simulink model "IEEE14_case"  (R2024b)
settings: Solver=FixedStepAuto  StartTime=0  StopTime=2  FixedStep=1e-7  RelTol=1e-3
values from neighbouring files (symbols this model uses):
  GFL_15_Bva = 0.009    [IEEE14_parameters.m]
  GFL_15_C_bus_pu = 7.179419    [IEEE14_parameters.m]
  GFL_15_f0 = 60    [IEEE14_parameters.m]
  GFL_15_I_id = 691.26967    [IEEE14_parameters.m]
  GFL_15_I_iq = 691.26967    [IEEE14_parameters.m]
  GFL_15_I_od = 45.2207    [IEEE14_parameters.m]
  GFL_15_I_oq = 45.2207    [IEEE14_parameters.m]
  GFL_15_I_pll = 0.78    [IEEE14_parameters.m]
  GFL_15_Kdi = 0.09    [IEEE14_parameters.m]
  GFL_15_Kdo = 0.9    [IEEE14_parameters.m]
  GFL_15_Kqi = 0.09    [IEEE14_parameters.m]
  GFL_15_Kqo = 0.9    [IEEE14_parameters.m]
  GFL_15_Lg_pu = 0.631447    [IEEE14_parameters.m]
  GFL_15_mode = 1    [IEEE14_parameters.m]
  GFL_15_P_id = 3.7166    [IEEE14_parameters.m]
  GFL_15_P_iq = 3.7166    [IEEE14_parameters.m]
  GFL_15_P_od = 0.4798    [IEEE14_parameters.m]
  GFL_15_P_oq = 0.4798    [IEEE14_parameters.m]
  GFL_15_P_pll = 290.42    [IEEE14_parameters.m]
  GFL_15_Qe_ref = 0.2    [IEEE14_parameters.m]
  GFL_15_Rg_pu = 0.024016    [IEEE14_parameters.m]
  GFL_15_Sbase = 1.000000e+4    (= 10000)    [IEEE14_parameters.m]
  GFL_15_Tdi = 0.01    [IEEE14_parameters.m]
  GFL_15_Tdo = 0.2    [IEEE14_parameters.m]
  GFL_15_Tqi = 0.01    [IEEE14_parameters.m]
  GFL_15_Tqo = 0.2    [IEEE14_parameters.m]
  GFL_15_Vbase = 380    [IEEE14_parameters.m]
  GFL_15_Vdc_ref = 1.011475    [IEEE14_parameters.m]
  GFL_15_Vdcbase = 700    [IEEE14_parameters.m]
  GFL_15_vq_ref = 0    [IEEE14_parameters.m]
  GFL_16_Bva = 0.002    [IEEE14_parameters.m]
  GFL_16_C_bus_pu = 7.179419    [IEEE14_parameters.m]
  GFL_16_f0 = 60    [IEEE14_parameters.m]
  GFL_16_I_id = 691.26967    [IEEE14_parameters.m]
  GFL_16_I_iq = 691.26967    [IEEE14_parameters.m]
  GFL_16_I_od = 45.2207    [IEEE14_parameters.m]
  GFL_16_I_oq = 45.2207    [IEEE14_parameters.m]
  GFL_16_I_pll = 0.78    [IEEE14_parameters.m]
  GFL_16_Kdi = 0.05    [IEEE14_parameters.m]
  GFL_16_Kdo = 0.5    [IEEE14_parameters.m]
  GFL_16_Kqi = 0.05    [IEEE14_parameters.m]
  GFL_16_Kqo = 0.5    [IEEE14_parameters.m]
  GFL_16_Lg_pu = 0.631447    [IEEE14_parameters.m]
  GFL_16_mode = 1    [IEEE14_parameters.m]
  GFL_16_P_id = 3.7166    [IEEE14_parameters.m]
  GFL_16_P_iq = 3.7166    [IEEE14_parameters.m]
  GFL_16_P_od = 0.4798    [IEEE14_parameters.m]
  GFL_16_P_oq = 0.4798    [IEEE14_parameters.m]
  GFL_16_P_pll = 290.42    [IEEE14_parameters.m]
  GFL_16_Qe_ref = 0.2    [IEEE14_parameters.m]
  GFL_16_Rg_pu = 0.024016    [IEEE14_parameters.m]
  GFL_16_Sbase = 1.000000e+4    (= 10000)    [IEEE14_parameters.m]
  GFL_16_Tdi = 0.01    [IEEE14_parameters.m]
  GFL_16_Tdo = 0.2    [IEEE14_parameters.m]
  GFL_16_Tqi = 0.01    [IEEE14_parameters.m]
  GFL_16_Tqo = 0.2    [IEEE14_parameters.m]
  GFL_16_Vbase = 380    [IEEE14_parameters.m]
  GFL_16_Vdc_ref = 1.01144    [IEEE14_parameters.m]
  GFL_16_Vdcbase = 700    [IEEE14_parameters.m]
  GFL_16_vq_ref = 0    [IEEE14_parameters.m]
  GFL_17_Bva = 0.002    [IEEE14_parameters.m]
  GFL_17_C_bus_pu = 7.179419    [IEEE14_parameters.m]
  GFL_17_f0 = 60    [IEEE14_parameters.m]
  GFL_17_I_id = 691.26967    [IEEE14_parameters.m]
  GFL_17_I_iq = 691.26967    [IEEE14_parameters.m]
  GFL_17_I_od = 45.2207    [IEEE14_parameters.m]
  GFL_17_I_oq = 45.2207    [IEEE14_parameters.m]
  GFL_17_I_pll = 0.78    [IEEE14_parameters.m]
  GFL_17_Kdi = 0.05    [IEEE14_parameters.m]
  GFL_17_Kdo = 0.5    [IEEE14_parameters.m]
  GFL_17_Kqi = 0.05    [IEEE14_parameters.m]
  GFL_17_Kqo = 0.5    [IEEE14_parameters.m]
  GFL_17_Lg_pu = 0.631447    [IEEE14_parameters.m]
  GFL_17_mode = 1    [IEEE14_parameters.m]
  GFL_17_P_id = 3.7166    [IEEE14_parameters.m]
  GFL_17_P_iq = 3.7166    [IEEE14_parameters.m]
  GFL_17_P_od = 0.4798    [IEEE14_parameters.m]
  GFL_17_P_oq = 0.4798    [IEEE14_parameters.m]
  GFL_17_P_pll = 290.42    [IEEE14_parameters.m]
  GFL_17_Qe_ref = 0.2    [IEEE14_parameters.m]
  GFL_17_Rg_pu = 0.024016    [IEEE14_parameters.m]
  GFL_17_Sbase = 1.000000e+4    (= 10000)    [IEEE14_parameters.m]
  GFL_17_Tdi = 0.01    [IEEE14_parameters.m]
  GFL_17_Tdo = 0.2    [IEEE14_parameters.m]
  GFL_17_Tqi = 0.01    [IEEE14_parameters.m]
  GFL_17_Tqo = 0.2    [IEEE14_parameters.m]
  GFL_17_Vbase = 380    [IEEE14_parameters.m]
  GFL_17_Vdc_ref = 1.011632    [IEEE14_parameters.m]
  GFL_17_Vdcbase = 700    [IEEE14_parameters.m]
  GFL_17_vq_ref = 0    [IEEE14_parameters.m]
  GFL_18_Bva = 0.002    [IEEE14_parameters.m]
  GFL_18_C_bus_pu = 7.179419    [IEEE14_parameters.m]
  GFL_18_f0 = 60    [IEEE14_parameters.m]
  GFL_18_I_id = 691.26967    [IEEE14_parameters.m]
  GFL_18_I_iq = 691.26967    [IEEE14_parameters.m]
  GFL_18_I_od = 45.2207    [IEEE14_parameters.m]
  GFL_18_I_oq = 45.2207    [IEEE14_parameters.m]
  GFL_18_I_pll = 0.78    [IEEE14_parameters.m]
  GFL_18_Kdi = 0.05    [IEEE14_parameters.m]
  GFL_18_Kdo = 0.5    [IEEE14_parameters.m]
  GFL_18_Kqi = 0.05    [IEEE14_parameters.m]
  GFL_18_Kqo = 0.5    [IEEE14_parameters.m]
  GFL_18_Lg_pu = 0.631447    [IEEE14_parameters.m]
  GFL_18_mode = 1    [IEEE14_parameters.m]
  GFL_18_P_id = 3.7166    [IEEE14_parameters.m]
  GFL_18_P_iq = 3.7166    [IEEE14_parameters.m]
  GFL_18_P_od = 0.4798    [IEEE14_parameters.m]
  GFL_18_P_oq = 0.4798    [IEEE14_parameters.m]
  GFL_18_P_pll = 290.42    [IEEE14_parameters.m]
  GFL_18_Qe_ref = 0.2    [IEEE14_parameters.m]
  GFL_18_Rg_pu = 0.024016    [IEEE14_parameters.m]
  GFL_18_Sbase = 1.000000e+4    (= 10000)    [IEEE14_parameters.m]
  GFL_18_Tdi = 0.01    [IEEE14_parameters.m]
  GFL_18_Tdo = 0.2    [IEEE14_parameters.m]
  GFL_18_Tqi = 0.01    [IEEE14_parameters.m]
  GFL_18_Tqo = 0.2    [IEEE14_parameters.m]
  GFL_18_Vbase = 380    [IEEE14_parameters.m]
  GFL_18_Vdc_ref = 1.011572    [IEEE14_parameters.m]
  GFL_18_Vdcbase = 700    [IEEE14_parameters.m]
  GFL_18_vq_ref = 0    [IEEE14_parameters.m]
  ... (+180 more)
(part 17 of 25)

== system IEEE14_case/SG_D_1/i_q_SG_D_1_block ==
  note: i_q_SG_D_1 in case14gfl
      | $-\frac{\sin\left(\theta _{\mathrm{SG},D,1}\right)\,\left(\psi _{q,\mathrm{SG},D,1}+\frac{\psi _{\mathrm{gq},\mathrm{SG},D,1}\,\left(x_{l}-x_{\mathrm{qdd}}\right)}{x_{l}-x_{\mathrm{qd}}}+\frac{\psi _{\mathrm{kq},\mathrm{SG},D,1}\,\left(x_{\mathrm{qd}}-x_{\mathrm{qdd}}\right)}{x_{l}-x_{\mathrm{qd}}}\right)}{x_{\mathrm{qdd}}}-\frac{\cos\left(\theta _{\mathrm{SG},D,1}\right)\,\left(\frac{\psi _{\mathrm{1d},\mathrm{SG},D,1}\,\left(x_{\mathrm{dd}}-x_{\mathrm{ddd}}\right)}{x_{\mathrm{dd}}-x_{l}}-\psi _{d,\mathrm{SG},D,1}+\frac{\psi _{\mathrm{fd},\mathrm{SG},D,1}\,\left(x_{\mathrm{ddd}}-x_{l}\right)}{x_{\mathrm{dd}}-x_{l}}\right)}{x_{\mathrm{ddd}}}$
      | Automatically generated on 2025-10-09 21:30:34 .
  State_psi_gq_SG_D_1_70f72 : Inport
  State_psi_kq_SG_D_1_fbc68 : Inport  Port=2
  State_psi_q_SG_D_1_42b5e : Inport  Port=3
  State_theta_SG_D_1_4335e : Inport  Port=4
  State_psi_1d_SG_D_1_63ddd : Inport  Port=5
  State_psi_d_SG_D_1_986bb : Inport  Port=6
  State_psi_fd_SG_D_1_ad572 : Inport  Port=7
  State_theta_SG_D_1_fd587 : Inport  Port=8
  Add_114d2 : Sum
  Add_45027 : Sum
  Add_56220 : Sum
  Add_ae113 : Sum
  Add_b9464 : Sum
  Add_b9521 : Sum
  Constant_-1_127fa : Constant  Value=-1
  Constant_-1_3da60 : Constant  Value=-1
  Constant_-1_73326 : Constant  Value=-1
  Constant_-1_a142a : Constant  Value=-1
  Constant_-1_edccd : Constant  Value=-1
  Constant_x_dd_58bf0 : Constant  Value=x_dd
  Constant_x_dd_5d4ff : Constant  Value=x_dd
  Constant_x_dd_82964 : Constant  Value=x_dd
  Constant_x_ddd_518ef : Constant  Value=x_ddd
  Constant_x_ddd_74ae2 : Constant  Value=x_ddd
  Constant_x_ddd_ec5d5 : Constant  Value=x_ddd
  Constant_x_l_24632 : Constant  Value=x_l
  Constant_x_l_71a65 : Constant  Value=x_l
  Constant_x_l_81874 : Constant  Value=x_l
  Constant_x_l_c732d : Constant  Value=x_l
  Constant_x_l_c7c9c : Constant  Value=x_l
  Constant_x_l_ee5e2 : Constant  Value=x_l
  Constant_x_qd_30086 : Constant  Value=x_qd
  Constant_x_qd_aec28 : Constant  Value=x_qd
  Constant_x_qd_b3788 : Constant  Value=x_qd
  Constant_x_qdd_5d370 : Constant  Value=x_qdd
  Constant_x_qdd_97975 : Constant  Value=x_qdd
  Constant_x_qdd_a11a2 : Constant  Value=x_qdd
  Divide_019c3 : Product  Inputs=*/
  Divide_537b6 : Product  Inputs=*/
  Divide_7faa8 : Product  Inputs=*/
  Divide_d8318 : Product  Inputs=*/
  Divide_edb7b : Product  Inputs=*/
  Divide_fddae : Product  Inputs=*/
  MathFunc_cos_33d3f : Trigonometry  Operator=cos
  MathFunc_sin_c8fbb : Trigonometry
  Product_1fa76 : Product
  Product_25a2e : Product
  Product_2e292 : Product
  Product_35172 : Product
  Product_5342a : Product
  Product_769ad : Product
  Product_9c475 : Product
  Product_afb73 : Product
  Product_b6c70 : Product
  Product_ccd5a : Product
  Product_e4bc8 : Product
  Subtract_0582b : Sum  Inputs=+-
  Subtract_2c857 : Sum  Inputs=+-
  Subtract_34bd0 : Sum  Inputs=+-
  Subtract_3512e : Sum  Inputs=+-
  Subtract_8240a : Sum  Inputs=+-
  Subtract_bada2 : Sum  Inputs=+-
  Subtract_e7035 : Sum  Inputs=+-
  Blockout_i_q_SG_D_1_04b1b : Outport
  wires:
  State_theta_SG_D_1_fd587/1 -> MathFunc_cos_33d3f/1
  State_psi_fd_SG_D_1_ad572/1 -> Product_25a2e/1
  Constant_-1_73326/1 -> Product_e4bc8/1
  Constant_x_l_71a65/1 -> Product_e4bc8/2
  Subtract_2c857/1 -> Product_25a2e/2
  Constant_x_l_24632/1 -> Subtract_8240a/2
  Product_e4bc8/1 -> Add_56220/1
  Constant_x_qdd_a11a2/1 -> Add_56220/2
  Constant_x_qd_30086/1 -> Subtract_e7035/1
  Constant_x_qdd_5d370/1 -> Divide_537b6/2
  MathFunc_sin_c8fbb/1 -> Product_1fa76/2
  Constant_-1_edccd/1 -> Product_b6c70/1
  Constant_x_qdd_97975/1 -> Subtract_e7035/2
  Add_ae113/1 -> Product_5342a/2
  Product_2e292/1 -> Divide_019c3/1
  Constant_x_l_c732d/1 -> Product_b6c70/2
  Constant_-1_a142a/1 -> Product_769ad/1
  Constant_x_l_ee5e2/1 -> Product_769ad/2
  State_psi_gq_SG_D_1_70f72/1 -> Product_2e292/1
  Add_56220/1 -> Product_2e292/2
  Divide_edb7b/1 -> Add_b9521/1
  Product_b6c70/1 -> Add_114d2/1
  Divide_537b6/1 -> Add_b9464/1
  Constant_x_qd_b3788/1 -> Add_114d2/2
  State_psi_kq_SG_D_1_fbc68/1 -> Product_9c475/1
  Add_b9521/1 -> Subtract_bada2/1
  Subtract_e7035/1 -> Product_9c475/2
  Divide_019c3/1 -> Subtract_3512e/1
  Add_114d2/1 -> Divide_019c3/2
  Product_769ad/1 -> Add_45027/1
  Constant_x_qd_aec28/1 -> Add_45027/2
  Constant_-1_127fa/1 -> Product_afb73/1
  MathFunc_cos_33d3f/1 -> Product_35172/2
  Product_25a2e/1 -> Divide_fddae/1
  State_psi_1d_SG_D_1_63ddd/1 -> Product_afb73/2
  Constant_x_l_c7c9c/1 -> Subtract_34bd0/2
  Constant_x_dd_58bf0/1 -> Subtract_0582b/1
  Divide_fddae/1 -> Subtract_bada2/2
  Constant_x_ddd_ec5d5/1 -> Subtract_0582b/2
  Product_35172/1 -> Divide_7faa8/1
  Product_9c475/1 -> Divide_d8318/1
  Product_afb73/1 -> Product_ccd5a/1
  Add_45027/1 -> Divide_d8318/2
  Subtract_0582b/1 -> Product_ccd5a/2
  State_psi_d_SG_D_1_986bb/1 -> Add_b9521/2
  Constant_x_dd_5d4ff/1 -> Subtract_8240a/1
  Constant_x_ddd_74ae2/1 -> Subtract_2c857/1
  Constant_x_l_81874/1 -> Subtract_2c857/2
  Divide_7faa8/1 -> Add_b9464/2
  Divide_d8318/1 -> Subtract_3512e/2
  State_theta_SG_D_1_4335e/1 -> MathFunc_sin_c8fbb/1
  Product_ccd5a/1 -> Divide_edb7b/1
  Subtract_8240a/1 -> Divide_edb7b/2
  Constant_x_dd_82964/1 -> Subtract_34bd0/1
  Subtract_3512e/1 -> Add_ae113/1
  State_psi_q_SG_D_1_42b5e/1 -> Add_ae113/2
  Subtract_34bd0/1 -> Divide_fddae/2
  Subtract_bada2/1 -> Product_35172/1
  Constant_-1_3da60/1 -> Product_5342a/1
  Product_5342a/1 -> Product_1fa76/1
  Product_1fa76/1 -> Divide_537b6/1
  Constant_x_ddd_518ef/1 -> Divide_7faa8/2
  Add_b9464/1 -> Blockout_i_q_SG_D_1_04b1b/1

== system IEEE14_case/SG_D_1/theta_SG_D_1_out_block ==
  note: theta_SG_D_1_out in case14gfl
      | $\theta _{\mathrm{SG},D,1}$
      | Automatically generated on 2025-10-09 21:30:39 .
  State_theta_SG_D_1_c8a88 : Inport
  Blockout_theta_SG_D_1_out_3d7c0 : Outport
  wires:
  State_theta_SG_D_1_c8a88/1 -> Blockout_theta_SG_D_1_out_3d7c0/1

== system IEEE14_case/SG_D_1/w_SG_D_1_out_block ==
  note: w_SG_D_1_out in case14gfl
      | $w_{\mathrm{SG},D,1}$
      | Automatically generated on 2025-10-09 21:30:39 .
  State_w_SG_D_1_b42d2 : Inport
  Blockout_w_SG_D_1_out_d4c3b : Outport
  wires:
  State_w_SG_D_1_b42d2/1 -> Blockout_w_SG_D_1_out_d4c3b/1

== system IEEE14_case/SG_D_2/T_e_SG_D_2_block ==
  note: T_e_SG_D_2 in case14gfl
      | $-\frac{\psi _{d,\mathrm{SG},D,2}\,\left(\psi _{q,\mathrm{SG},D,2}+\frac{\psi _{\mathrm{gq},\mathrm{SG},D,2}\,\left(x_{l}-x_{\mathrm{qdd}}\right)}{x_{l}-x_{\mathrm{qd}}}+\frac{\psi _{\mathrm{kq},\mathrm{SG},D,2}\,\left(x_{\mathrm{qd}}-x_{\mathrm{qdd}}\right)}{x_{l}-x_{\mathrm{qd}}}\right)}{x_{\mathrm{qdd}}}-\frac{\psi _{q,\mathrm{SG},D,2}\,\left(\frac{\psi _{\mathrm{1d},\mathrm{SG},D,2}\,\left(x_{\mathrm{dd}}-x_{\mathrm{ddd}}\right)}{x_{\mathrm{dd}}-x_{l}}-\psi _{d,\mathrm{SG},D,2}+\frac{\psi _{\mathrm{fd},\mathrm{SG},D,2}\,\left(x_{\mathrm{ddd}}-x_{l}\right)}{x_{\mathrm{dd}}-x_{l}}\right)}{x_{\mathrm{ddd}}}$
      | Automatically generated on 2025-10-09 21:31:38 .
  State_psi_d_SG_D_2_5317f : Inport
  State_psi_gq_SG_D_2_6936d : Inport  Port=2
  State_psi_kq_SG_D_2_8eee7 : Inport  Port=3
  State_psi_q_SG_D_2_7be04 : Inport  Port=4
  State_psi_q_SG_D_2_caf2c : Inport  Port=5
  State_psi_1d_SG_D_2_2fd39 : Inport  Port=6
  State_psi_d_SG_D_2_ed23a : Inport  Port=7
  State_psi_fd_SG_D_2_ca537 : Inport  Port=8
  Add_2b3c2 : Sum
  Add_688ad : Sum
  Add_696f2 : Sum
  Add_c50cf : Sum
  Add_ca6b5 : Sum
  Add_da9df : Sum
  Constant_-1_1cd99 : Constant  Value=-1
  Constant_-1_4d652 : Constant  Value=-1
  Constant_-1_79bb3 : Constant  Value=-1
  Constant_-1_d53d8 : Constant  Value=-1
  Constant_-1_f498c : Constant  Value=-1
  Constant_x_dd_7815d : Constant  Value=x_dd
  Constant_x_dd_aa8f8 : Constant  Value=x_dd
  Constant_x_dd_b97d0 : Constant  Value=x_dd
  Constant_x_ddd_1ce26 : Constant  Value=x_ddd
  Constant_x_ddd_af070 : Constant  Value=x_ddd
  Constant_x_ddd_b27d2 : Constant  Value=x_ddd
  Constant_x_l_60110 : Constant  Value=x_l
  Constant_x_l_8205c : Constant  Value=x_l
  Constant_x_l_ada53 : Constant  Value=x_l
  Constant_x_l_c73fb : Constant  Value=x_l
  Constant_x_l_c8c4d : Constant  Value=x_l
  Constant_x_l_d282e : Constant  Value=x_l
  Constant_x_qd_3426f : Constant  Value=x_qd
  Constant_x_qd_a4aa5 : Constant  Value=x_qd
  Constant_x_qd_afc2c : Constant  Value=x_qd
  Constant_x_qdd_8196f : Constant  Value=x_qdd
  Constant_x_qdd_85b1a : Constant  Value=x_qdd
  Constant_x_qdd_9702e : Constant  Value=x_qdd
  Divide_40679 : Product  Inputs=*/
  Divide_9391f : Product  Inputs=*/
  Divide_a4479 : Product  Inputs=*/
  Divide_b1adc : Product  Inputs=*/
  Divide_ce550 : Product  Inputs=*/
  Divide_f2e46 : Product  Inputs=*/
  Product_0284d : Product
  Product_03e58 : Product
  Product_0976d : Product
  Product_18365 : Product
  Product_18539 : Product
  Product_42b56 : Product
  Product_842de : Product
  Product_8e0ef : Product
  Product_93504 : Product
  Product_bb7e4 : Product
  Product_ffa4d : Product
  Subtract_0a39a : Sum  Inputs=+-
  Subtract_33ab6 : Sum  Inputs=+-
  Subtract_37d77 : Sum  Inputs=+-
  Subtract_39521 : Sum  Inputs=+-
  Subtract_7bb21 : Sum  Inputs=+-
  Subtract_8f489 : Sum  Inputs=+-
  Subtract_9bdb1 : Sum  Inputs=+-
  Blockout_T_e_SG_D_2_7a393 : Outport
  wires:
  Constant_-1_1cd99/1 -> Product_18365/1
  Divide_f2e46/1 -> Subtract_33ab6/1
  Constant_-1_f498c/1 -> Product_03e58/1
  Constant_x_l_8205c/1 -> Product_03e58/2
  Constant_x_qd_a4aa5/1 -> Subtract_39521/1
  Product_18539/1 -> Divide_f2e46/1
  Product_03e58/1 -> Add_696f2/1
  Divide_40679/1 -> Subtract_37d77/2
  Constant_x_qdd_85b1a/1 -> Subtract_39521/2
  Constant_x_qdd_8196f/1 -> Divide_9391f/2
  Constant_x_ddd_b27d2/1 -> Subtract_9bdb1/2
  Constant_x_qdd_9702e/1 -> Add_696f2/2
  Constant_x_l_c8c4d/1 -> Product_18365/2
  Constant_-1_d53d8/1 -> Product_842de/1
  Constant_x_l_c73fb/1 -> Product_842de/2
  Constant_-1_79bb3/1 -> Product_0284d/1
  State_psi_1d_SG_D_2_2fd39/1 -> Product_0284d/2
  Constant_x_dd_b97d0/1 -> Subtract_9bdb1/1
  Divide_b1adc/1 -> Subtract_33ab6/2
  State_psi_gq_SG_D_2_6936d/1 -> Product_18539/1
  Add_696f2/1 -> Product_18539/2
  Subtract_33ab6/1 -> Add_ca6b5/1
  Constant_x_dd_7815d/1 -> Subtract_7bb21/1
  Product_18365/1 -> Add_688ad/1
  Product_0976d/1 -> Product_93504/1
  Constant_x_qd_3426f/1 -> Add_688ad/2
  State_psi_kq_SG_D_2_8eee7/1 -> Product_42b56/1
  Subtract_39521/1 -> Product_42b56/2
  Product_842de/1 -> Add_c50cf/1
  State_psi_q_SG_D_2_caf2c/1 -> Product_8e0ef/1
  Constant_x_qd_afc2c/1 -> Add_c50cf/2
  Product_0284d/1 -> Product_ffa4d/1
  Divide_a4479/1 -> Add_2b3c2/2
  Subtract_9bdb1/1 -> Product_ffa4d/2
  Constant_x_l_60110/1 -> Subtract_7bb21/2
  Constant_x_ddd_1ce26/1 -> Subtract_0a39a/1
  Constant_x_dd_aa8f8/1 -> Subtract_8f489/1
  Constant_x_l_d282e/1 -> Subtract_0a39a/2
  Add_2b3c2/1 -> Blockout_T_e_SG_D_2_7a393/1
  Add_688ad/1 -> Divide_f2e46/2
  Product_42b56/1 -> Divide_b1adc/1
  Product_93504/1 -> Divide_9391f/1
  State_psi_d_SG_D_2_5317f/1 -> Product_0976d/2
  Add_c50cf/1 -> Divide_b1adc/2
  Product_ffa4d/1 -> Divide_ce550/1
  Subtract_7bb21/1 -> Divide_ce550/2
  Constant_x_l_ada53/1 -> Subtract_8f489/2
  State_psi_fd_SG_D_2_ca537/1 -> Product_bb7e4/1
  Constant_x_ddd_af070/1 -> Divide_a4479/2
  Product_8e0ef/1 -> Divide_a4479/1
  Subtract_0a39a/1 -> Product_bb7e4/2
  Divide_ce550/1 -> Add_da9df/1
  State_psi_d_SG_D_2_ed23a/1 -> Add_da9df/2
  Add_da9df/1 -> Subtract_37d77/1
  Product_bb7e4/1 -> Divide_40679/1
  Subtract_8f489/1 -> Divide_40679/2
  Constant_-1_4d652/1 -> Product_0976d/1
  State_psi_q_SG_D_2_7be04/1 -> Add_ca6b5/2
  Add_ca6b5/1 -> Product_93504/2
  Subtract_37d77/1 -> Product_8e0ef/2
  Divide_9391f/1 -> Add_2b3c2/1

== system IEEE14_case/SG_D_2/d_E_fd_SG_D_2_block ==
  note: d_E_fd_SG_D_2 in case14gfl
      | $\frac{V_{f,\mathrm{SG},D,2}-E_{\mathrm{fd},\mathrm{SG},D,2}\,K_{E}}{T_{E}}$
      | Automatically generated on 2025-10-09 21:31:24 .
  State_E_fd_SG_D_2_0281f : Inport
  State_V_f_SG_D_2_6e69e : Inport  Port=2
  Add_e3f49 : Sum
  Constant_-1_30831 : Constant  Value=-1
  Constant_K_E_1b384 : Constant  Value=K_E
  Constant_T_E_17208 : Constant  Value=T_E
  Divide_cf4a7 : Product  Inputs=*/
  Product_d4c8e : Product
  Product_f9e82 : Product
  Blockout_d_E_fd_SG_D_2_3931e : Outport
  wires:
  Constant_-1_30831/1 -> Product_f9e82/1
  State_E_fd_SG_D_2_0281f/1 -> Product_f9e82/2
  Product_f9e82/1 -> Product_d4c8e/1
  Constant_K_E_1b384/1 -> Product_d4c8e/2
  Product_d4c8e/1 -> Add_e3f49/1
  Constant_T_E_17208/1 -> Divide_cf4a7/2
  State_V_f_SG_D_2_6e69e/1 -> Add_e3f49/2
  Add_e3f49/1 -> Divide_cf4a7/1
  Divide_cf4a7/1 -> Blockout_d_E_fd_SG_D_2_3931e/1

== system IEEE14_case/SG_D_2/d_Px_1_SG_D_2_block ==
  note: d_Px_1_SG_D_2 in case14gfl
      | $\frac{w_{\mathrm{SG},D,2}-2\,\pi \,f_{0}}{T_{w}}-\frac{\mathrm{Px}_{1,\mathrm{SG},D,2}}{T_{w}}$
      | Automatically generated on 2025-10-09 21:31:25 .
  State_Px_1_SG_D_2_416e3 : Inport
  State_w_SG_D_2_57c67 : Inport  Port=2
  Add_551aa : Sum
  Add_9ff0d : Sum
  Constant_-1_98426 : Constant  Value=-1
  Constant_-2.0_b655b : Constant  Value=-2.0
  Constant_T_w_ad641 : Constant  Value=T_w
  Constant_T_w_ce180 : Constant  Value=T_w
  Constant_f0_10368 : Constant  Value=f0
  Constant_pi_95a6b : Constant  Value=pi
  Divide_44d16 : Product  Inputs=*/
  Divide_d2f91 : Product  Inputs=*/
  Product_1d3f0 : Product
  Product_6c5f2 : Product
  Product_d4b45 : Product
  Blockout_d_Px_1_SG_D_2_466a7 : Outport
  wires:
  Constant_-2.0_b655b/1 -> Product_d4b45/1
  State_w_SG_D_2_57c67/1 -> Add_551aa/2
  Constant_pi_95a6b/1 -> Product_d4b45/2
  Product_d4b45/1 -> Product_6c5f2/1
  Constant_f0_10368/1 -> Product_6c5f2/2
  Constant_-1_98426/1 -> Product_1d3f0/1
  State_Px_1_SG_D_2_416e3/1 -> Product_1d3f0/2
  Product_6c5f2/1 -> Add_551aa/1
  Product_1d3f0/1 -> Divide_d2f91/1
  Constant_T_w_ce180/1 -> Divide_d2f91/2
  Add_551aa/1 -> Divide_44d16/1
  Constant_T_w_ad641/1 -> Divide_44d16/2
  Divide_d2f91/1 -> Add_9ff0d/1
  Divide_44d16/1 -> Add_9ff0d/2
  Add_9ff0d/1 -> Blockout_d_Px_1_SG_D_2_466a7/1

== system IEEE14_case/SG_D_2/d_Px_2_SG_D_2_block ==
  note: d_Px_2_SG_D_2 in case14gfl
      | $\frac{\mathrm{Px}_{1,\mathrm{SG},D,2}-T_{2}\,\left(\frac{\mathrm{Px}_{1,\mathrm{SG},D,2}}{T_{w}}-\frac{w_{\mathrm{SG},D,2}-2\,\pi \,f_{0}}{T_{w}}\right)}{T_{1}}-\frac{\mathrm{Px}_{2,\mathrm{SG},D,2}}{T_{1}}$
      | Automatically generated on 2025-10-09 21:31:26 .
  State_Px_2_SG_D_2_863da : Inport
  State_Px_1_SG_D_2_cbeb2 : Inport  Port=2
  State_Px_1_SG_D_2_01235 : Inport  Port=3
  State_w_SG_D_2_0c27f : Inport  Port=4
  Add_a434e : Sum
  Add_a5257 : Sum
  Add_c47ed : Sum
  Add_c6eb0 : Sum
  Constant_-1_5e988 : Constant  Value=-1
  Constant_-1_b1f8a : Constant  Value=-1
  Constant_-2.0_39250 : Constant  Value=-2.0
  Constant_T_1_3104f : Constant  Value=T_1
  Constant_T_1_e5327 : Constant  Value=T_1
  Constant_T_2_9ff96 : Constant  Value=T_2
  Constant_T_w_01571 : Constant  Value=T_w
  Constant_T_w_3c3a1 : Constant  Value=T_w
  Constant_f0_1ecf9 : Constant  Value=f0
  Constant_pi_4ae66 : Constant  Value=pi
  Divide_505a9 : Product  Inputs=*/
  Divide_677ae : Product  Inputs=*/
  Divide_c07f0 : Product  Inputs=*/
  Divide_e4026 : Product  Inputs=*/
  Product_33552 : Product
  Product_36a8c : Product
  Product_412bc : Product
  Product_a9983 : Product
  Product_b475d : Product
  Blockout_d_Px_2_SG_D_2_dd680 : Outport
  wires:
  Constant_-1_5e988/1 -> Product_a9983/1
  Constant_-2.0_39250/1 -> Product_33552/1
  Product_412bc/1 -> Add_a5257/2
  State_w_SG_D_2_0c27f/1 -> Add_c6eb0/2
  Constant_pi_4ae66/1 -> Product_33552/2
  Product_33552/1 -> Product_36a8c/1
  State_Px_1_SG_D_2_01235/1 -> Product_b475d/2
  Constant_f0_1ecf9/1 -> Product_36a8c/2
  State_Px_2_SG_D_2_863da/1 -> Product_a9983/2
  Constant_-1_b1f8a/1 -> Product_b475d/1
  Product_36a8c/1 -> Add_c6eb0/1
  Product_b475d/1 -> Divide_505a9/1
  Constant_T_w_3c3a1/1 -> Divide_505a9/2
  Add_c6eb0/1 -> Divide_c07f0/1
  Constant_T_w_01571/1 -> Divide_c07f0/2
  Divide_505a9/1 -> Add_c47ed/1
  Divide_c07f0/1 -> Add_c47ed/2
  Constant_T_2_9ff96/1 -> Product_412bc/1
  Add_c47ed/1 -> Product_412bc/2
  State_Px_1_SG_D_2_cbeb2/1 -> Add_a5257/1
  Product_a9983/1 -> Divide_e4026/1
  Constant_T_1_e5327/1 -> Divide_e4026/2
  Add_a5257/1 -> Divide_677ae/1
  Constant_T_1_3104f/1 -> Divide_677ae/2
  Divide_e4026/1 -> Add_a434e/1
  Divide_677ae/1 -> Add_a434e/2
  Add_a434e/1 -> Blockout_d_Px_2_SG_D_2_dd680/1

== system IEEE14_case/SG_D_2/d_Px_3_SG_D_2_block ==
  note: d_Px_3_SG_D_2 in case14gfl
      | $\frac{\mathrm{Px}_{2,\mathrm{SG},D,2}+T_{4}\,\left(\frac{\mathrm{Px}_{1,\mathrm{SG},D,2}-T_{2}\,\left(\frac{\mathrm{Px}_{1,\mathrm{SG},D,2}}{T_{w}}-\frac{w_{\mathrm{SG},D,2}-2\,\pi \,f_{0}}{T_{w}}\right)}{T_{1}}-\frac{\mathrm{Px}_{2,\mathrm{SG},D,2}}{T_{1}}\right)}{T_{3}}-\frac{\mathrm{Px}_{3,\mathrm{SG},D,2}}{T_{3}}$
      | Automatically generated on 2025-10-09 21:31:28 .
  State_Px_3_SG_D_2_18957 : Inport
  State_Px_2_SG_D_2_b3dc6 : Inport  Port=2
  State_Px_2_SG_D_2_577d6 : Inport  Port=3
  State_Px_1_SG_D_2_b7377 : Inport  Port=4
  State_Px_1_SG_D_2_616ef : Inport  Port=5
  State_w_SG_D_2_29f15 : Inport  Port=6
  Add_22d1e : Sum
  Add_2d414 : Sum
  Add_39c98 : Sum
  Add_a3176 : Sum
  Add_f1115 : Sum
  Add_fad9b : Sum
  Constant_-1_5ae8e : Constant  Value=-1
  Constant_-1_b7761 : Constant  Value=-1
  Constant_-1_c8859 : Constant  Value=-1
  Constant_-2.0_4440b : Constant  Value=-2.0
  Constant_T_1_77873 : Constant  Value=T_1
  Constant_T_1_e4b78 : Constant  Value=T_1
  Constant_T_2_bd3ce : Constant  Value=T_2
  Constant_T_3_0300b : Constant  Value=T_3
  Constant_T_3_75dad : Constant  Value=T_3
  Constant_T_4_2c8ce : Constant  Value=T_4
  Constant_T_w_77fd9 : Constant  Value=T_w
  Constant_T_w_a773b : Constant  Value=T_w
  Constant_f0_da9a7 : Constant  Value=f0
  Constant_pi_3b5bc : Constant  Value=pi
  Divide_10e03 : Product  Inputs=*/
  Divide_11950 : Product  Inputs=*/
  Divide_4cdcd : Product  Inputs=*/
  Divide_5a835 : Product  Inputs=*/
  Divide_89948 : Product  Inputs=*/
  Divide_a4b2b : Product  Inputs=*/
  Product_390e7 : Product
  Product_64aa0 : Product
  Product_7ff1c : Product
  Product_a0410 : Product
  Product_d624a : Product
  Product_d74e4 : Product
  Product_ee4eb : Product
  Blockout_d_Px_3_SG_D_2_c9fb9 : Outport
  wires:
  Constant_-2.0_4440b/1 -> Product_7ff1c/1
  State_w_SG_D_2_29f15/1 -> Add_a3176/2
  Add_f1115/1 -> Divide_a4b2b/1
  Constant_pi_3b5bc/1 -> Product_7ff1c/2
  Constant_-1_c8859/1 -> Product_390e7/1
  Product_7ff1c/1 -> Product_d74e4/1
  State_Px_2_SG_D_2_577d6/1 -> Product_390e7/2
  State_Px_1_SG_D_2_616ef/1 -> Product_ee4eb/2
  Divide_a4b2b/1 -> Add_39c98/2
  Constant_f0_da9a7/1 -> Product_d74e4/2
  Constant_-1_b7761/1 -> Product_ee4eb/1
  Product_d74e4/1 -> Add_a3176/1
  Product_ee4eb/1 -> Divide_5a835/1
  Constant_T_w_a773b/1 -> Divide_5a835/2
  Divide_4cdcd/1 -> Add_39c98/1
  Add_a3176/1 -> Divide_10e03/1
  Product_a0410/1 -> Add_2d414/2
  Constant_T_w_77fd9/1 -> Divide_10e03/2
  Divide_5a835/1 -> Add_fad9b/1
  State_Px_1_SG_D_2_b7377/1 -> Add_2d414/1
  Divide_10e03/1 -> Add_fad9b/2
  Constant_-1_5ae8e/1 -> Product_d624a/1
  Constant_T_2_bd3ce/1 -> Product_a0410/1
  Add_fad9b/1 -> Product_a0410/2
  Product_390e7/1 -> Divide_89948/1
  Constant_T_1_e4b78/1 -> Divide_89948/2
  Add_2d414/1 -> Divide_11950/1
  Constant_T_1_77873/1 -> Divide_11950/2
  Divide_89948/1 -> Add_22d1e/1
  Divide_11950/1 -> Add_22d1e/2
  Constant_T_4_2c8ce/1 -> Product_64aa0/1
  Add_22d1e/1 -> Product_64aa0/2
  State_Px_3_SG_D_2_18957/1 -> Product_d624a/2
  State_Px_2_SG_D_2_b3dc6/1 -> Add_f1115/1
  Product_64aa0/1 -> Add_f1115/2
  Product_d624a/1 -> Divide_4cdcd/1
  Constant_T_3_0300b/1 -> Divide_4cdcd/2
  Constant_T_3_75dad/1 -> Divide_a4b2b/2
  Add_39c98/1 -> Blockout_d_Px_3_SG_D_2_c9fb9/1

== system IEEE14_case/SG_D_2/d_R_f_SG_D_2_block ==
  note: d_R_f_SG_D_2 in case14gfl
      | $-\frac{R_{f,\mathrm{SG},D,2}-\frac{E_{\mathrm{fd},\mathrm{SG},D,2}\,K_{F}}{T_{F}}}{T_{F}}$
      | Automatically generated on 2025-10-09 21:31:23 .
  State_E_fd_SG_D_2_d9efc : Inport
  State_R_f_SG_D_2_a3c1e : Inport  Port=2
  Constant_K_F_06d49 : Constant  Value=K_F
  Constant_T_F_64c31 : Constant  Value=T_F
  Constant_T_F_86413 : Constant  Value=T_F
  Divide_33dc5 : Product  Inputs=*/
  Divide_98bc2 : Product  Inputs=*/
  Product_dd782 : Product
  Subtract_efc4a : Sum  Inputs=+-
  Blockout_d_R_f_SG_D_2_1f586 : Outport
  wires:
  Constant_T_F_86413/1 -> Divide_98bc2/2
  State_E_fd_SG_D_2_d9efc/1 -> Product_dd782/1
  Constant_K_F_06d49/1 -> Product_dd782/2
  State_R_f_SG_D_2_a3c1e/1 -> Subtract_efc4a/2
  Product_dd782/1 -> Divide_98bc2/1
  Divide_98bc2/1 -> Subtract_efc4a/1
  Constant_T_F_64c31/1 -> Divide_33dc5/2
  Subtract_efc4a/1 -> Divide_33dc5/1
  Divide_33dc5/1 -> Blockout_d_R_f_SG_D_2_1f586/1

== system IEEE14_case/SG_D_2/d_T_m_SG_D_2_block ==
  note: d_T_m_SG_D_2 in case14gfl
      | $-\frac{T_{m,\mathrm{SG},D,2}-T_{0}+\frac{\mathrm{SpeedPara}\,\left(w_{\mathrm{SG},D,2}-w_{\mathrm{ref}}\right)}{2\,f_{0}\,\pi }}{T_{\mathrm{speed}}}$
      | Automatically generated on 2025-10-09 21:31:15 .
  State_w_SG_D_2_28412 : Inport
  State_T_m_SG_D_2_839d4 : Inport  Port=2
  Add_1b156 : Sum
  Add_22663 : Sum
  Constant_-1_6e153 : Constant  Value=-1
  Constant_2.0_9b3af : Constant  Value=2.0
  Constant_SpeedPara_2246e : Constant  Value=SpeedPara
  Constant_T_0_ef356 : Constant  Value=T_0
  Constant_T_speed_16b8d : Constant  Value=T_speed
  Constant_f0_898be : Constant  Value=f0
  Constant_pi_3a176 : Constant  Value=pi
  Constant_w_ref_d87f4 : Constant  Value=w_ref
  Divide_8fee5 : Product  Inputs=*/
  Divide_dafba : Product  Inputs=*/
  Product_86f03 : Product
  Product_8ef4b : Product
  Product_9a3b8 : Product
  Product_f325b : Product
  Subtract_935fb : Sum  Inputs=+-
  Blockout_d_T_m_SG_D_2_a859c : Outport
  wires:
  Constant_pi_3a176/1 -> Product_8ef4b/2
  Constant_-1_6e153/1 -> Product_f325b/1
  Constant_w_ref_d87f4/1 -> Add_22663/2
  State_w_SG_D_2_28412/1 -> Product_f325b/2
  Product_f325b/1 -> Add_22663/1
  Add_1b156/1 -> Subtract_935fb/1
  Add_22663/1 -> Product_9a3b8/2
  Constant_2.0_9b3af/1 -> Product_8ef4b/1
  Constant_SpeedPara_2246e/1 -> Product_9a3b8/1
  Product_8ef4b/1 -> Product_86f03/1
  Constant_f0_898be/1 -> Product_86f03/2
  Product_9a3b8/1 -> Divide_8fee5/1
  Product_86f03/1 -> Divide_8fee5/2
  Divide_8fee5/1 -> Add_1b156/1
  Constant_T_0_ef356/1 -> Add_1b156/2
  State_T_m_SG_D_2_839d4/1 -> Subtract_935fb/2
  Subtract_935fb/1 -> Divide_dafba/1
  Constant_T_speed_16b8d/1 -> Divide_dafba/2
  Divide_dafba/1 -> Blockout_d_T_m_SG_D_2_a859c/1

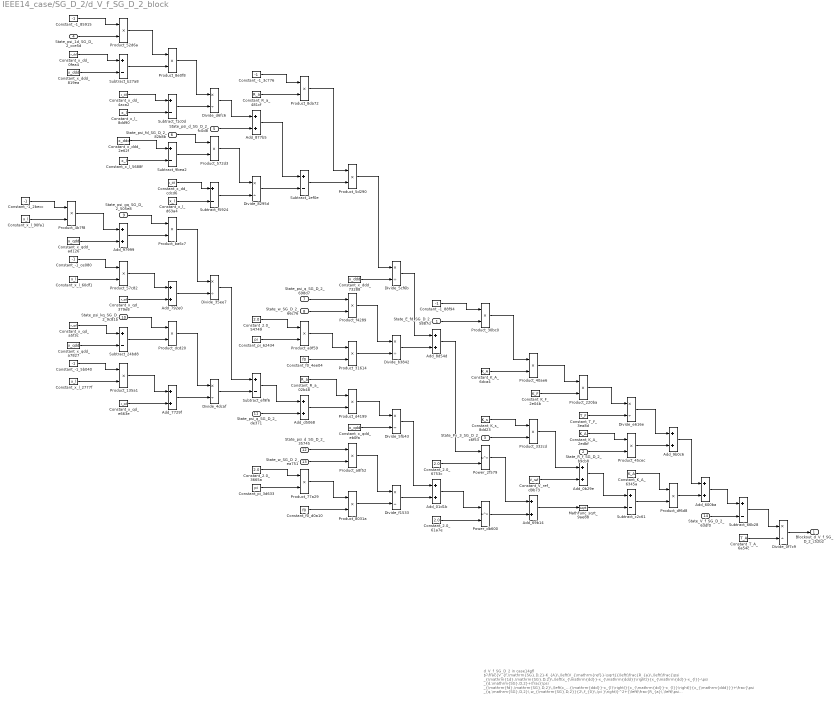
== system IEEE14_case/SG_D_2/d_V_f_SG_D_2_block ==
  note: d_V_f_SG_D_2 in case14gfl
      | $-\frac{V_{f,\mathrm{SG},D,2}-K_{A}\,\left(V_{\mathrm{ref}}-\sqrt{{\left(\frac{R_{a}\,\left(\frac{\psi _{\mathrm{1d},\mathrm{SG},D,2}\,\left(x_{\mathrm{dd}}-x_{\mathrm{ddd}}\right)}{x_{\mathrm{dd}}-x_{l}}-\psi _{d,\mathrm{SG},D,2}+\frac{\psi _{\mathrm{fd},\mathrm{SG},D,2}\,\left(x_{\mathrm{ddd}}-x_{l}\right)}{x_{\mathrm{dd}}-x_{l}}\right)}{x_{\mathrm{ddd}}}+\frac{\psi _{q,\mathrm{SG},D,2}\,w_{\mathrm{SG},D,2}}{2\,f_{0}\,\pi }\right)}^2+{\left(\frac{R_{a}\,\left(\psi _{q,\mathrm{SG},D,2}+\frac{\psi _{\mathrm{gq},\mathrm{SG},D,2}\,\left(x_{l}-x_{\mathrm{qdd}}\right)}{x_{l}-x_{\mathrm{qd}}}+\frac{\psi _{\mathrm{kq},\mathrm{SG},D,2}\,\left(x_{\mathrm{qd}}-x_{\mathrm{qdd}}\right)}{x_{l}-x_{\mathrm{qd}}}\right)}{x_{\mathrm{qdd}}}+\frac{\psi _{d,\mathrm{SG},D,2}\,w_{\mathrm{SG},D,2}}{2\,f_{0}\,\pi }\right)}^2}+K_{s}\,\mathrm{Px}_{3,\mathrm{SG},D,2}\right)-K_{A}\,R_{f,\mathrm{SG},D,2}+\frac{E_{\mathrm{fd},\mathrm{SG},D,2}\,K_{A}\,K_{F}}{T_{F}}}{T_{A}}$
      | Automatically generated on 2025-10-09 21:31:21 .
  State_E_fd_SG_D_2_5887d : Inport
  State_R_f_SG_D_2_b9cb8 : Inport  Port=2
  State_Px_3_SG_D_2_c6f53 : Inport  Port=3
  State_psi_1d_SG_D_2_cce5d : Inport  Port=4
  State_psi_d_SG_D_2_fc0d8 : Inport  Port=5
  State_psi_fd_SG_D_2_82b8b : Inport  Port=6
  State_psi_q_SG_D_2_698d7 : Inport  Port=7
  State_w_SG_D_2_66c76 : Inport  Port=8
  State_psi_gq_SG_D_2_505e8 : Inport  Port=9
  State_psi_kq_SG_D_2_9c81b : Inport  Port=10
  State_psi_q_SG_D_2_de371 : Inport  Port=11
  State_psi_d_SG_D_2_35745 : Inport  Port=12
  State_w_SG_D_2_ea751 : Inport  Port=13
  State_V_f_SG_D_2_63df0 : Inport  Port=14
  Add_01d1b : Sum
  Add_0b29e : Sum
  Add_600ba : Sum
  Add_69b14 : Sum
  Add_7729f : Sum
  Add_792e0 : Sum
  Add_877b5 : Sum
  Add_8d54d : Sum
  Add_97999 : Sum
  Add_9b0c6 : Sum
  Add_d5068 : Sum
  Constant_-1_2becc : Constant  Value=-1
  Constant_-1_3c776 : Constant  Value=-1
  Constant_-1_5b040 : Constant  Value=-1
  Constant_-1_85915 : Constant  Value=-1
  Constant_-1_88f94 : Constant  Value=-1
  Constant_-1_ce080 : Constant  Value=-1
  Constant_2.0_3665a : Constant  Value=2.0
  Constant_2.0_54749 : Constant  Value=2.0
  Constant_2.0_61a7e : Constant  Value=2.0
  Constant_2.0_6753c : Constant  Value=2.0
  Constant_K_A_2edbf : Constant  Value=K_A
  Constant_K_A_6345a : Constant  Value=K_A
  Constant_K_A_6dca4 : Constant  Value=K_A
  Constant_K_F_2e04b : Constant  Value=K_F
  Constant_K_s_8dd23 : Constant  Value=K_s
  Constant_R_a_02b48 : Constant  Value=R_a
  Constant_R_a_481cf : Constant  Value=R_a
  Constant_T_A_6a54c : Constant  Value=T_A
  Constant_T_F_3ea8d : Constant  Value=T_F
  Constant_V_ref_d9b73 : Constant  Value=V_ref
  Constant_f0_4ee04 : Constant  Value=f0
  Constant_f0_d0a10 : Constant  Value=f0
  Constant_pi_3d633 : Constant  Value=pi
  Constant_pi_62434 : Constant  Value=pi
  Constant_x_dd_0fea4 : Constant  Value=x_dd
  Constant_x_dd_4aca2 : Constant  Value=x_dd
  Constant_x_dd_cdcd6 : Constant  Value=x_dd
  Constant_x_ddd_2e62f : Constant  Value=x_ddd
  Constant_x_ddd_73288 : Constant  Value=x_ddd
  Constant_x_ddd_819ea : Constant  Value=x_ddd
  Constant_x_l_2777f : Constant  Value=x_l
  Constant_x_l_5688f : Constant  Value=x_l
  Constant_x_l_60df1 : Constant  Value=x_l
  Constant_x_l_8dd90 : Constant  Value=x_l
  Constant_x_l_90fa1 : Constant  Value=x_l
  Constant_x_l_d63a4 : Constant  Value=x_l
  Constant_x_qd_379e8 : Constant  Value=x_qd
  Constant_x_qd_a5f3c : Constant  Value=x_qd
  Constant_x_qd_e663e : Constant  Value=x_qd
  Constant_x_qdd_a7827 : Constant  Value=x_qdd
  Constant_x_qdd_ad126 : Constant  Value=x_qdd
  Constant_x_qdd_eb0fa : Constant  Value=x_qdd
  Divide_0f7c9 : Product  Inputs=*/
  Divide_35ee7 : Product  Inputs=*/
  Divide_4dcaf : Product  Inputs=*/
  Divide_5cf6b : Product  Inputs=*/
  Divide_5fb43 : Product  Inputs=*/
  Divide_8295d : Product  Inputs=*/
  Divide_b3842 : Product  Inputs=*/
  Divide_d6fc6 : Product  Inputs=*/
  Divide_e616e : Product  Inputs=*/
  Divide_f1533 : Product  Inputs=*/
  MathFunc_sqrt_9ae88 : Sqrt
  Power_2f579 : Math  Operator=pow
  Power_db600 : Math  Operator=pow
  Product_135a1 : Product
  Product_220ba : Product
  Product_30bc0 : Product
  Product_31614 : Product
  Product_332cd : Product
  Product_40ae6 : Product
  Product_45cec : Product
  Product_4b7f8 : Product
  Product_52d6a : Product
  Product_572d3 : Product
  Product_57c82 : Product
  Product_5d290 : Product
  Product_77a29 : Product
  Product_8031a : Product
  Product_8da72 : Product
  Product_8e0f8 : Product
  Product_a8f52 : Product
  Product_a9f59 : Product
  Product_ba6c7 : Product
  Product_d4199 : Product
  Product_dcd20 : Product
  Product_df6d8 : Product
  Product_f4289 : Product
  Subtract_1ef0e : Sum  Inputs=+-
  Subtract_24bd8 : Sum  Inputs=+-
  Subtract_66b28 : Sum  Inputs=+-
  Subtract_9bea2 : Sum  Inputs=+-
  Subtract_b27a8 : Sum  Inputs=+-
  Subtract_c2c61 : Sum  Inputs=+-
  Subtract_ef9f6 : Sum  Inputs=+-
  Subtract_f1c0d : Sum  Inputs=+-
  Subtract_f5924 : Sum  Inputs=+-
  Blockout_d_V_f_SG_D_2_c52b2 : Outport
  wires:
  Constant_-1_85915/1 -> Product_52d6a/1
  Constant_2.0_54749/1 -> Product_a9f59/1
  Constant_-1_2becc/1 -> Product_4b7f8/1
  Product_a9f59/1 -> Product_31614/1
  Product_4b7f8/1 -> Add_97999/1
  Constant_x_l_2777f/1 -> Product_135a1/2
  Constant_x_l_90fa1/1 -> Product_4b7f8/2
  State_psi_1d_SG_D_2_cce5d/1 -> Product_52d6a/2
  Constant_x_l_d63a4/1 -> Subtract_f5924/2
  Constant_x_dd_0fea4/1 -> Subtract_b27a8/1
  Product_d4199/1 -> Divide_5fb43/1
  Constant_x_ddd_819ea/1 -> Subtract_b27a8/2
  Constant_x_qd_e663e/1 -> Add_7729f/2
  Add_97999/1 -> Product_ba6c7/2
  Constant_x_qdd_ad126/1 -> Add_97999/2
  Constant_-1_ce080/1 -> Product_57c82/1
  Constant_x_dd_cdcd6/1 -> Subtract_f5924/1
  Subtract_ef9f6/1 -> Add_d5068/1
  Power_2f579/1 -> Add_69b14/1
  Constant_x_l_60df1/1 -> Product_57c82/2
  Constant_2.0_3665a/1 -> Product_77a29/1
  Constant_x_qd_a5f3c/1 -> Subtract_24bd8/1
  Constant_pi_3d633/1 -> Product_77a29/2
  Subtract_1ef0e/1 -> Product_5d290/2
  Constant_x_qdd_a7827/1 -> Subtract_24bd8/2
  State_psi_fd_SG_D_2_82b8b/1 -> Product_572d3/1
  Constant_-1_5b040/1 -> Product_135a1/1
  Product_52d6a/1 -> Product_8e0f8/1
  State_w_SG_D_2_ea751/1 -> Product_a8f52/2
  Subtract_b27a8/1 -> Product_8e0f8/2
  Constant_x_dd_4aca2/1 -> Subtract_f1c0d/1
  State_psi_q_SG_D_2_de371/1 -> Add_d5068/2
  State_w_SG_D_2_66c76/1 -> Product_f4289/2
  Subtract_9bea2/1 -> Product_572d3/2
  Constant_x_l_8dd90/1 -> Subtract_f1c0d/2
  Add_9b0c6/1 -> Add_600ba/1
  Constant_x_ddd_2e62f/1 -> Subtract_9bea2/1
  Constant_x_l_5688f/1 -> Subtract_9bea2/2
  State_psi_gq_SG_D_2_505e8/1 -> Product_ba6c7/1
  Product_57c82/1 -> Add_792e0/1
  Subtract_f5924/1 -> Divide_8295d/2
  Constant_x_qd_379e8/1 -> Add_792e0/2
  Product_f4289/1 -> Divide_b3842/1
  State_psi_kq_SG_D_2_9c81b/1 -> Product_dcd20/1
  Subtract_24bd8/1 -> Product_dcd20/2
  Product_572d3/1 -> Divide_8295d/1
  State_V_f_SG_D_2_63df0/1 -> Subtract_66b28/2
  Product_135a1/1 -> Add_7729f/1
  Product_8e0f8/1 -> Divide_d6fc6/1
  Divide_35ee7/1 -> Subtract_ef9f6/1
  Subtract_f1c0d/1 -> Divide_d6fc6/2
  Product_ba6c7/1 -> Divide_35ee7/1
  Add_792e0/1 -> Divide_35ee7/2
  Product_dcd20/1 -> Divide_4dcaf/1
  Divide_8295d/1 -> Subtract_1ef0e/2
  Constant_f0_4ee04/1 -> Product_31614/2
  Add_7729f/1 -> Divide_4dcaf/2
  Divide_d6fc6/1 -> Add_877b5/1
  State_psi_d_SG_D_2_fc0d8/1 -> Add_877b5/2
  Divide_4dcaf/1 -> Subtract_ef9f6/2
  Constant_-1_3c776/1 -> Product_8da72/1
  Constant_R_a_481cf/1 -> Product_8da72/2
  Constant_f0_d0a10/1 -> Product_8031a/2
  Add_877b5/1 -> Subtract_1ef0e/1
  Product_8da72/1 -> Product_5d290/1
  Constant_pi_62434/1 -> Product_a9f59/2
  State_psi_q_SG_D_2_698d7/1 -> Product_f4289/1
  Constant_R_a_02b48/1 -> Product_d4199/1
  State_E_fd_SG_D_2_5887d/1 -> Product_30bc0/2
  Add_d5068/1 -> Product_d4199/2
  State_psi_d_SG_D_2_35745/1 -> Product_a8f52/1
  Product_77a29/1 -> Product_8031a/1
  Product_5d290/1 -> Divide_5cf6b/1
  Constant_x_ddd_73288/1 -> Divide_5cf6b/2
  Product_31614/1 -> Divide_b3842/2
  Constant_x_qdd_eb0fa/1 -> Divide_5fb43/2
  Product_a8f52/1 -> Divide_f1533/1
  Product_8031a/1 -> Divide_f1533/2
  Divide_5cf6b/1 -> Add_8d54d/1
  Divide_b3842/1 -> Add_8d54d/2
  Divide_5fb43/1 -> Add_01d1b/1
  Divide_f1533/1 -> Add_01d1b/2
  Constant_-1_88f94/1 -> Product_30bc0/1
  Add_8d54d/1 -> Power_2f579/1
  Constant_2.0_6753c/1 -> Power_2f579/2
  Add_01d1b/1 -> Power_db600/1
  Constant_2.0_61a7e/1 -> Power_db600/2
  Product_30bc0/1 -> Product_40ae6/1
  Constant_K_A_6dca4/1 -> Product_40ae6/2
  Constant_K_s_8dd23/1 -> Product_332cd/1
  State_Px_3_SG_D_2_c6f53/1 -> Product_332cd/2
  Power_db600/1 -> Add_69b14/2
  Product_40ae6/1 -> Product_220ba/1
  Constant_K_F_2e04b/1 -> Product_220ba/2
  Product_332cd/1 -> Add_0b29e/1
  Constant_V_ref_d9b73/1 -> Add_0b29e/2
  Add_69b14/1 -> MathFunc_sqrt_9ae88/1
  Product_220ba/1 -> Divide_e616e/1
  Constant_T_F_3ea8d/1 -> Divide_e616e/2
  Constant_K_A_2edbf/1 -> Product_45cec/1
  State_R_f_SG_D_2_b9cb8/1 -> Product_45cec/2
  Add_0b29e/1 -> Subtract_c2c61/1
  MathFunc_sqrt_9ae88/1 -> Subtract_c2c61/2
  Divide_e616e/1 -> Add_9b0c6/1
  Product_45cec/1 -> Add_9b0c6/2
  Constant_K_A_6345a/1 -> Product_df6d8/1
  Subtract_c2c61/1 -> Product_df6d8/2
  Product_df6d8/1 -> Add_600ba/2
  Add_600ba/1 -> Subtract_66b28/1
  Subtract_66b28/1 -> Divide_0f7c9/1
  Constant_T_A_6a54c/1 -> Divide_0f7c9/2
  Divide_0f7c9/1 -> Blockout_d_V_f_SG_D_2_c52b2/1

== system IEEE14_case/SG_D_2/d_psi_1d_SG_D_2_block ==
  note: d_psi_1d_SG_D_2 in case14gfl
      | $-\frac{\psi _{\mathrm{1d},\mathrm{SG},D,2}-\psi _{\mathrm{fd},\mathrm{SG},D,2}+\frac{\left(x_{\mathrm{dd}}-x_{l}\right)\,\left(\frac{\psi _{\mathrm{1d},\mathrm{SG},D,2}\,\left(x_{\mathrm{dd}}-x_{\mathrm{ddd}}\right)}{x_{\mathrm{dd}}-x_{l}}-\psi _{d,\mathrm{SG},D,2}+\frac{\psi _{\mathrm{fd},\mathrm{SG},D,2}\,\left(x_{\mathrm{ddd}}-x_{l}\right)}{x_{\mathrm{dd}}-x_{l}}\right)}{x_{\mathrm{ddd}}}}{T_{\mathrm{ddd}}}$
      | Automatically generated on 2025-10-09 21:31:00 .
  State_psi_1d_SG_D_2_5768c : Inport
  State_psi_fd_SG_D_2_4ee86 : Inport  Port=2
  State_psi_1d_SG_D_2_34f10 : Inport  Port=3
  State_psi_d_SG_D_2_f297a : Inport  Port=4
  State_psi_fd_SG_D_2_c105c : Inport  Port=5
  Add_41ee4 : Sum
  Add_49c58 : Sum
  Add_dba5c : Sum
  Constant_-1_25802 : Constant  Value=-1
  Constant_-1_7c223 : Constant  Value=-1
  Constant_T_ddd_5684f : Constant  Value=T_ddd
  Constant_x_dd_13f0a : Constant  Value=x_dd
  Constant_x_dd_1696b : Constant  Value=x_dd
  Constant_x_dd_21a68 : Constant  Value=x_dd
  Constant_x_dd_d73dc : Constant  Value=x_dd
  Constant_x_ddd_1b5ab : Constant  Value=x_ddd
  Constant_x_ddd_34eb7 : Constant  Value=x_ddd
  Constant_x_ddd_ccfbe : Constant  Value=x_ddd
  Constant_x_l_15d89 : Constant  Value=x_l
  Constant_x_l_16344 : Constant  Value=x_l
  Constant_x_l_a8c3c : Constant  Value=x_l
  Constant_x_l_bf11e : Constant  Value=x_l
  Divide_0f850 : Product  Inputs=*/
  Divide_2858e : Product  Inputs=*/
  Divide_b272e : Product  Inputs=*/
  Divide_e03d3 : Product  Inputs=*/
  Product_0c0f8 : Product
  Product_1784b : Product
  Product_232f3 : Product
  Product_29907 : Product
  Product_cb8af : Product
  Subtract_1e85e : Sum  Inputs=+-
  Subtract_28d8a : Sum  Inputs=+-
  Subtract_65b68 : Sum  Inputs=+-
  Subtract_c5429 : Sum  Inputs=+-
  Subtract_d49d7 : Sum  Inputs=+-
  Subtract_e1bbf : Sum  Inputs=+-
  Blockout_d_psi_1d_SG_D_2_81873 : Outport
  wires:
  Subtract_1e85e/1 -> Product_0c0f8/2
  Constant_x_l_15d89/1 -> Subtract_c5429/2
  Divide_2858e/1 -> Add_dba5c/2
  Subtract_28d8a/1 -> Product_232f3/2
  Constant_-1_7c223/1 -> Product_1784b/1
  Constant_x_dd_1696b/1 -> Subtract_d49d7/1
  Divide_e03d3/1 -> Blockout_d_psi_1d_SG_D_2_81873/1
  State_psi_fd_SG_D_2_4ee86/1 -> Add_41ee4/2
  State_psi_1d_SG_D_2_34f10/1 -> Product_1784b/2
  Divide_b272e/1 -> Subtract_28d8a/2
  Constant_x_ddd_34eb7/1 -> Subtract_d49d7/2
  State_psi_1d_SG_D_2_5768c/1 -> Product_29907/2
  Product_1784b/1 -> Product_cb8af/1
  Subtract_d49d7/1 -> Product_cb8af/2
  Constant_x_dd_13f0a/1 -> Subtract_c5429/1
  Constant_x_ddd_ccfbe/1 -> Subtract_1e85e/1
  Constant_x_l_a8c3c/1 -> Subtract_1e85e/2
  Product_cb8af/1 -> Divide_0f850/1
  Subtract_c5429/1 -> Divide_0f850/2
  State_psi_fd_SG_D_2_c105c/1 -> Product_0c0f8/1
  Constant_x_dd_21a68/1 -> Subtract_e1bbf/1
  Constant_x_l_bf11e/1 -> Subtract_65b68/2
  Constant_x_l_16344/1 -> Subtract_e1bbf/2
  Constant_x_ddd_1b5ab/1 -> Divide_2858e/2
  Divide_0f850/1 -> Add_49c58/1
  State_psi_d_SG_D_2_f297a/1 -> Add_49c58/2
  Product_0c0f8/1 -> Divide_b272e/1
  Subtract_e1bbf/1 -> Divide_b272e/2
  Constant_x_dd_d73dc/1 -> Subtract_65b68/1
  Add_49c58/1 -> Subtract_28d8a/1
  Constant_-1_25802/1 -> Product_29907/1
  Subtract_65b68/1 -> Product_232f3/1
  Product_29907/1 -> Add_41ee4/1
  Product_232f3/1 -> Divide_2858e/1
  Add_41ee4/1 -> Add_dba5c/1
  Add_dba5c/1 -> Divide_e03d3/1
  Constant_T_ddd_5684f/1 -> Divide_e03d3/2

== system IEEE14_case/SG_D_2/d_psi_d_SG_D_2_block ==
  note: d_psi_d_SG_D_2 in case14gfl
      | $2\,\pi \,f_{0}\,\left(v_{d,\mathrm{SG},D,2}\,\sin\left(\theta _{\mathrm{SG},D,2}\right)-v_{q,\mathrm{SG},D,2}\,\cos\left(\theta _{\mathrm{SG},D,2}\right)+\frac{R_{a}\,\left(\frac{\psi _{\mathrm{1d},\mathrm{SG},D,2}\,\left(x_{\mathrm{dd}}-x_{\mathrm{ddd}}\right)}{x_{\mathrm{dd}}-x_{l}}-\psi _{d,\mathrm{SG},D,2}+\frac{\psi _{\mathrm{fd},\mathrm{SG},D,2}\,\left(x_{\mathrm{ddd}}-x_{l}\right)}{x_{\mathrm{dd}}-x_{l}}\right)}{x_{\mathrm{ddd}}}+\frac{\psi _{q,\mathrm{SG},D,2}\,w_{\mathrm{SG},D,2}}{2\,f_{0}\,\pi }\right)$
      | Automatically generated on 2025-10-09 21:30:50 .
  State_psi_1d_SG_D_2_d5455 : Inport
  State_psi_d_SG_D_2_46d33 : Inport  Port=2
  State_psi_fd_SG_D_2_e734d : Inport  Port=3
  Input_v_d_SG_D_2_d6dc0 : Inport  Port=4
  State_theta_SG_D_2_fba08 : Inport  Port=5
  Input_v_q_SG_D_2_00db2 : Inport  Port=6
  State_theta_SG_D_2_1738b : Inport  Port=7
  State_psi_q_SG_D_2_54a7c : Inport  Port=8
  State_w_SG_D_2_3bf29 : Inport  Port=9
  Add_3d3b0 : Sum
  Add_512e6 : Sum
  Constant_-1_a926b : Constant  Value=-1
  Constant_-2.0_72ddd : Constant  Value=-2.0
  Constant_2.0_fd6cc : Constant  Value=2.0
  Constant_R_a_f013e : Constant  Value=R_a
  Constant_f0_1bc02 : Constant  Value=f0
  Constant_f0_dba99 : Constant  Value=f0
  Constant_pi_89608 : Constant  Value=pi
  Constant_pi_cbbcb : Constant  Value=pi
  Constant_x_dd_1013f : Constant  Value=x_dd
  Constant_x_dd_10e60 : Constant  Value=x_dd
  Constant_x_dd_e28c0 : Constant  Value=x_dd
  Constant_x_ddd_71aa8 : Constant  Value=x_ddd
  Constant_x_ddd_cea58 : Constant  Value=x_ddd
  Constant_x_ddd_d6dc2 : Constant  Value=x_ddd
  Constant_x_l_1ab87 : Constant  Value=x_l
  Constant_x_l_39597 : Constant  Value=x_l
  Constant_x_l_7db23 : Constant  Value=x_l
  Divide_39735 : Product  Inputs=*/
  Divide_c3797 : Product  Inputs=*/
  Divide_dfea9 : Product  Inputs=*/
  Divide_ef280 : Product  Inputs=*/
  MathFunc_cos_92f86 : Trigonometry  Operator=cos
  MathFunc_sin_55757 : Trigonometry
  Product_11c1e : Product
  Product_4c68d : Product
  Product_4dc8e : Product
  Product_5da53 : Product
  Product_97e26 : Product
  Product_a0da5 : Product
  Product_a8613 : Product
  Product_abe9c : Product
  Product_b77be : Product
  Product_c191d : Product
  Product_e758e : Product
  Product_f0c43 : Product
  Subtract_1c799 : Sum  Inputs=+-
  Subtract_31f93 : Sum  Inputs=+-
  Subtract_4ae03 : Sum  Inputs=+-
  Subtract_60c59 : Sum  Inputs=+-
  Subtract_78d11 : Sum  Inputs=+-
  Subtract_a9603 : Sum  Inputs=+-
  Subtract_e5501 : Sum  Inputs=+-
  Blockout_d_psi_d_SG_D_2_bb4d6 : Outport
  wires:
  MathFunc_sin_55757/1 -> Product_4c68d/2
  Constant_x_dd_10e60/1 -> Subtract_60c59/1
  Constant_-1_a926b/1 -> Product_97e26/1
  Constant_x_l_39597/1 -> Subtract_60c59/2
  State_psi_1d_SG_D_2_d5455/1 -> Product_97e26/2
  Constant_f0_1bc02/1 -> Product_11c1e/2
  Constant_2.0_fd6cc/1 -> Product_a0da5/1
  Constant_x_l_7db23/1 -> Subtract_e5501/2
  Constant_x_dd_e28c0/1 -> Subtract_4ae03/1
  Product_a8613/1 -> Blockout_d_psi_d_SG_D_2_bb4d6/1
  Constant_pi_cbbcb/1 -> Product_a0da5/2
  Constant_x_ddd_cea58/1 -> Subtract_4ae03/2
  Subtract_1c799/1 -> Product_a8613/2
  Product_97e26/1 -> Product_b77be/1
  Product_a0da5/1 -> Product_abe9c/1
  Subtract_4ae03/1 -> Product_b77be/2
  Divide_ef280/1 -> Subtract_1c799/2
  Constant_x_ddd_d6dc2/1 -> Subtract_78d11/1
  Constant_x_l_1ab87/1 -> Subtract_78d11/2
  Product_b77be/1 -> Divide_c3797/1
  Subtract_31f93/1 -> Add_512e6/1
  Subtract_60c59/1 -> Divide_c3797/2
  State_psi_fd_SG_D_2_e734d/1 -> Product_f0c43/1
  Subtract_78d11/1 -> Product_f0c43/2
  Constant_x_dd_1013f/1 -> Subtract_e5501/1
  Divide_c3797/1 -> Add_3d3b0/1
  State_psi_d_SG_D_2_46d33/1 -> Add_3d3b0/2
  Product_f0c43/1 -> Divide_39735/1
  Subtract_e5501/1 -> Divide_39735/2
  Add_3d3b0/1 -> Subtract_a9603/1
  Divide_39735/1 -> Subtract_a9603/2
  Constant_R_a_f013e/1 -> Product_4dc8e/1
  Subtract_a9603/1 -> Product_4dc8e/2
  Divide_dfea9/1 -> Subtract_31f93/1
  State_theta_SG_D_2_fba08/1 -> MathFunc_sin_55757/1
  Product_4dc8e/1 -> Divide_dfea9/1
  Constant_-2.0_72ddd/1 -> Product_e758e/1
  Input_v_d_SG_D_2_d6dc0/1 -> Product_4c68d/1
  Constant_x_ddd_71aa8/1 -> Divide_dfea9/2
  State_theta_SG_D_2_1738b/1 -> MathFunc_cos_92f86/1
  Product_11c1e/1 -> Product_a8613/1
  Product_4c68d/1 -> Subtract_31f93/2
  Product_e758e/1 -> Product_11c1e/1
  Input_v_q_SG_D_2_00db2/1 -> Product_c191d/1
  MathFunc_cos_92f86/1 -> Product_c191d/2
  State_psi_q_SG_D_2_54a7c/1 -> Product_5da53/1
  State_w_SG_D_2_3bf29/1 -> Product_5da53/2
  Constant_f0_dba99/1 -> Product_abe9c/2
  Constant_pi_89608/1 -> Product_e758e/2
  Product_c191d/1 -> Add_512e6/2
  Product_5da53/1 -> Divide_ef280/1
  Product_abe9c/1 -> Divide_ef280/2
  Add_512e6/1 -> Subtract_1c799/1
